simulink model "GFLIB_AtanYX_BAM_F16"  (Simulink 8.3)
settings: Solver=ode45  StartTime=0.0  StopTime=10.0  RelTol=1e-3
settings Model: Creator=RE004C  LastModifiedBy=B17364
settings OptimizationCC: ExpressionDepthLimit=2147483647
settings DebuggingCC: FcnCallInpInsideContextMsg=UseLocalSettings  StrictBusMsg=Warning
settings HardwareCC: ProdLargestAtomicInteger=Long  ProdLargestAtomicFloat=Double  ProdIntDivRoundTo=Zero  ProdEndianess=BigEndian  ProdHWDeviceType=Freescale->32-bit PowerPC

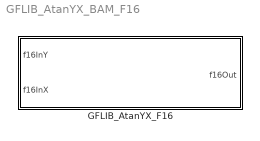
== system GFLIB_AtanYX_BAM_F16 ==
  GFLIB_AtanYX_F16 : Subsystem  mask(GFLIB_AtanYX_F16){}
      mask help: Bit accurate model of GFLIB_AtanYX function.
      mask init:
      | pos = get_param(gcb, 'Position');width = pos(3) - pos(1); height = pos(4) - pos(2);tX=width/2;tY=height*0.9;
      mask Display: color('black');port_label('input',1,'f16InY');port_label('input',2,'f16InX');port_label('output',1,'f16Out');color('black');disp('GFLIB_AtanYX_F16');color('blue');text(tX,tY, 'BAM', 'horizontalAlignment', 'center');

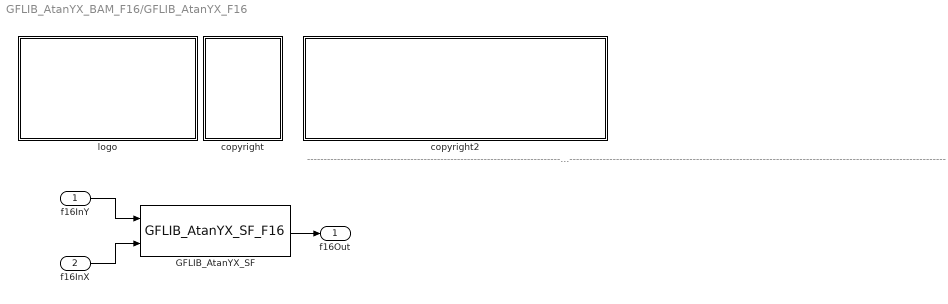
== system GFLIB_AtanYX_BAM_F16/GFLIB_AtanYX_F16 ==
  note: ---------------------------------------------------------------------------------------------------------------------------------------------------------------------------------------------------
  f16InY : Inport
  f16InX : Inport  Port=2
  GFLIB_AtanYX_SF : S-Function  FunctionName=GFLIB_AtanYX_SF_F16  EnableBusSupport=off
  copyright : Subsystem
      mask Display:
      | text(10,90,'FILE:');text(10,75,'DESRIPTION:')
      | text(10,60,'COPYRIGHT:')
      | text(10,45,'VERSION:')
      | text(10,30,'DATE:')
  copyright2 : Subsystem
      mask Display:
      | text(10,90,'GFLIB_AtanYX_BAM_F16.mdl');text(10,75,'YX Arctangent of argument.');text(10,60,'Freescale')
      | text(10,45,'0.1');text(10,30,'05-Sep-2011');
  logo : Subsystem
      mask Display: image(imread('logo.jpg'))
  f16Out : Outport
  wires:
  f16InY/1 -> GFLIB_AtanYX_SF/1
  f16InX/1 -> GFLIB_AtanYX_SF/2
  GFLIB_AtanYX_SF/1 -> f16Out/1

== system GFLIB_AtanYX_BAM_F16/GFLIB_AtanYX_F16/copyright ==

== system GFLIB_AtanYX_BAM_F16/GFLIB_AtanYX_F16/copyright2 ==

== system GFLIB_AtanYX_BAM_F16/GFLIB_AtanYX_F16/logo ==
